simulink library "tenneco_lib"  (R2016b)
settings: Solver=ode45  StartTime=0.0  StopTime=10.0  RelTol=1e-3
undefined symbols (not defined in the file): Com_cntAMBInitTO_c, Com_cntAMBStopTO_c, Com_cntEC1InitTO_c, Com_cntEC1StopTO_c, Com_swAMBRx_c, Com_swEC1Rx_c, Com_swUseSPN108_c, Com_swUseSPN543_c, const, Env_pAmbPDflt_c, Env_pAmbPKOff_c, Env_pAmbPOvrd_c, Env_swAmbPOvrd_c, MSG_INIT_TIMEOUT, MSG_NOT_RECEIVED, MSG_RECEIVED_NOW, MSG_STOP_TIMEOUT
libraries: simulink x19, tenneco_lib x2
(part 4 of 5)

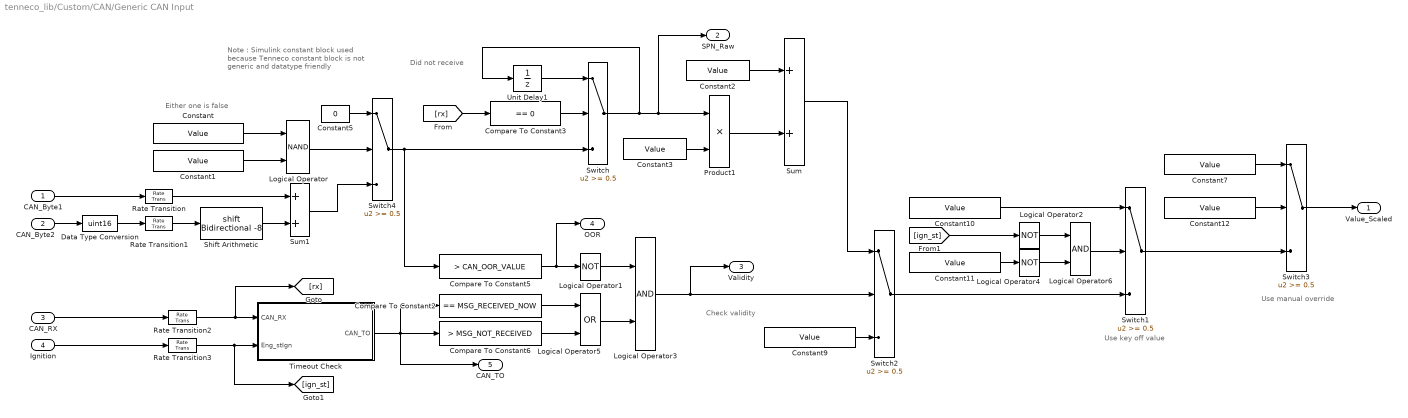
== system tenneco_lib/Custom/CAN/Generic CAN Input ==
  note: Either one is false
  note: Did not receive
  note: Use manual override
  note: Check validity
  note: Use key off value
  note: Note : Simulink constant block used because Tenneco constant block is not generic and datatype friendly
  CAN_Byte1 : Inport  mask(Standard Inport){Port=1}
      mask prompts: Port "Simulink:blkprm_prompts:InOutportPortNum"
      mask help: Provide an input port for subsystems.
      mask TypeOptions Port: Port
  CAN_Byte2 : Inport  Port=2  mask(Standard Inport){Port=2}
      mask prompts: Port "Simulink:blkprm_prompts:InOutportPortNum"
      mask help: Provide an input port for subsystems.
      mask TypeOptions Port: Port
  CAN_RX : Inport  Port=3  mask(Standard Inport){Port=3}
      mask prompts: Port "Simulink:blkprm_prompts:InOutportPortNum"
      mask help: Provide an input port for subsystems.
      mask TypeOptions Port: Port
  Ignition : Inport  Port=4  mask(Standard Inport){Port=4}
      mask prompts: Port "Simulink:blkprm_prompts:InOutportPortNum"
      mask help: Provide an input port for subsystems.
      mask TypeOptions Port: Port
  Compare To Constant2 : simulink/Logic and Bit Operations/Compare To Constant  relop===  const=MSG_RECEIVED_NOW  OutDataTypeStr=boolean
  Compare To Constant3 : simulink/Logic and Bit Operations/Compare To Constant  relop===  const=0  OutDataTypeStr=boolean
  Compare To Constant5 : simulink/Logic and Bit Operations/Compare To Constant  relop=>  const=CAN_OOR_VALUE  OutDataTypeStr=boolean
  Compare To Constant6 : simulink/Logic and Bit Operations/Compare To Constant  relop=>  const=MSG_NOT_RECEIVED  OutDataTypeStr=boolean
  Constant : Constant  Value=Value  mask(Constant){Value=CAN_USE_SW}
      mask prompts: Value "Simulink:blkprm_prompts:ConstConstValue"
      mask help: Output the constant specified by the 'Constant value' parameter. If 'Constant value' is a vector, treat the constant value as a 1-D array.
      mask init: same as tenneco_lib/Sources/Constant
      mask TypeOptions Value: Value
      mask Display: disp(str)
  Constant1 : Constant  Value=Value  mask(Constant){Value=CAN_RECV_SW}
      mask prompts: Value "Simulink:blkprm_prompts:ConstConstValue"
      mask help: Output the constant specified by the 'Constant value' parameter. If 'Constant value' is a vector, treat the constant value as a 1-D array.
      mask init: same as tenneco_lib/Sources/Constant
      mask TypeOptions Value: Value
      mask Display: disp(str)
  Constant10 : Constant  Value=Value  mask(Constant){Value=KEY_OFF_VALUE}
      mask prompts: Value "Simulink:blkprm_prompts:ConstConstValue"
      mask help: Output the constant specified by the 'Constant value' parameter. If 'Constant value' is a vector, treat the constant value as a 1-D array.
      mask init: same as tenneco_lib/Sources/Constant
      mask TypeOptions Value: Value
      mask Display: disp(str)
  Constant11 : Constant  Value=Value  mask(Constant){Value=MAN_OVRD_SW}
      mask prompts: Value "Simulink:blkprm_prompts:ConstConstValue"
      mask help: Output the constant specified by the 'Constant value' parameter. If 'Constant value' is a vector, treat the constant value as a 1-D array.
      mask init: same as tenneco_lib/Sources/Constant
      mask TypeOptions Value: Value
      mask Display: disp(str)
  Constant12 : Constant  Value=Value  mask(Constant){Value=MAN_OVRD_SW}
      mask prompts: Value "Simulink:blkprm_prompts:ConstConstValue"
      mask help: Output the constant specified by the 'Constant value' parameter. If 'Constant value' is a vector, treat the constant value as a 1-D array.
      mask init: same as tenneco_lib/Sources/Constant
      mask TypeOptions Value: Value
      mask Display: disp(str)
  Constant2 : Constant  Value=Value  mask(Constant){Value=OFFSET}
      mask prompts: Value "Simulink:blkprm_prompts:ConstConstValue"
      mask help: Output the constant specified by the 'Constant value' parameter. If 'Constant value' is a vector, treat the constant value as a 1-D array.
      mask init: same as tenneco_lib/Sources/Constant
      mask TypeOptions Value: Value
      mask Display: disp(str)
  Constant3 : Constant  Value=Value  mask(Constant){Value=SLOPE}
      mask prompts: Value "Simulink:blkprm_prompts:ConstConstValue"
      mask help: Output the constant specified by the 'Constant value' parameter. If 'Constant value' is a vector, treat the constant value as a 1-D array.
      mask init: same as tenneco_lib/Sources/Constant
      mask TypeOptions Value: Value
      mask Display: disp(str)
  Constant5 : Constant  Value=0  OutDataTypeStr=Inherit: Inherit via back propagation
  Constant7 : Constant  Value=Value  mask(Constant){Value=MAN_OVRD_VALUE}
      mask prompts: Value "Simulink:blkprm_prompts:ConstConstValue"
      mask help: Output the constant specified by the 'Constant value' parameter. If 'Constant value' is a vector, treat the constant value as a 1-D array.
      mask init: same as tenneco_lib/Sources/Constant
      mask TypeOptions Value: Value
      mask Display: disp(str)
  Constant9 : Constant  Value=Value  mask(Constant){Value=DEFAULT_VALUE}
      mask prompts: Value "Simulink:blkprm_prompts:ConstConstValue"
      mask help: Output the constant specified by the 'Constant value' parameter. If 'Constant value' is a vector, treat the constant value as a 1-D array.
      mask init: same as tenneco_lib/Sources/Constant
      mask TypeOptions Value: Value
      mask Display: disp(str)
  Data Type Conversion : DataTypeConversion  OutDataTypeStr=uint16  mask(Data Type Conversion){OutDataTypeStr=uint16}
      mask prompts: OutDataTypeStr "Simulink:blkprm_prompts:OUTPUT_UNIFIEDDATATYPE"
      mask help: Convert the input to the data type and scaling of the output.
      mask TypeOptions OutDataTypeStr: OutDataTypeStr
  Logical Operator : Logic  Operator=NAND  Inputs=Inputs  AllPortsSameDT=off  OutDataTypeStr=boolean  mask(Logical Operator){Operator=NAND, Inputs=2}
      mask prompts: Operator "Simulink:blkprm_prompts:LogicOperator"; Inputs "Simulink:blkprm_prompts:LogicNumInputPorts"
      mask help: Logical operators. For a single input, operators are applied across the input vector. For multiple inputs, operators are applied across the inputs.
      mask TypeOptions Operator: Operator
      mask TypeOptions Inputs: Inputs
  Logical Operator1 : Logic  Operator=NOT  Inputs=Inputs  AllPortsSameDT=off  OutDataTypeStr=boolean  mask(Logical Operator){Operator=NOT, Inputs=2}
      mask prompts: Operator "Simulink:blkprm_prompts:LogicOperator"; Inputs "Simulink:blkprm_prompts:LogicNumInputPorts"
      mask help: Logical operators. For a single input, operators are applied across the input vector. For multiple inputs, operators are applied across the inputs.
      mask TypeOptions Operator: Operator
      mask TypeOptions Inputs: Inputs
  Logical Operator2 : Logic  Operator=NOT  Inputs=Inputs  AllPortsSameDT=off  OutDataTypeStr=boolean  mask(Logical Operator){Operator=NOT, Inputs=2}
      mask prompts: Operator "Simulink:blkprm_prompts:LogicOperator"; Inputs "Simulink:blkprm_prompts:LogicNumInputPorts"
      mask help: Logical operators. For a single input, operators are applied across the input vector. For multiple inputs, operators are applied across the inputs.
      mask TypeOptions Operator: Operator
      mask TypeOptions Inputs: Inputs
  Logical Operator3 : Logic  Inputs=Inputs  AllPortsSameDT=off  OutDataTypeStr=boolean  mask(Logical Operator){Operator=AND, Inputs=2}
      mask prompts: Operator "Simulink:blkprm_prompts:LogicOperator"; Inputs "Simulink:blkprm_prompts:LogicNumInputPorts"
      mask help: Logical operators. For a single input, operators are applied across the input vector. For multiple inputs, operators are applied across the inputs.
      mask TypeOptions Operator: Operator
      mask TypeOptions Inputs: Inputs
  Logical Operator4 : Logic  Operator=NOT  Inputs=Inputs  AllPortsSameDT=off  OutDataTypeStr=boolean  mask(Logical Operator){Operator=NOT, Inputs=2}
      mask prompts: Operator "Simulink:blkprm_prompts:LogicOperator"; Inputs "Simulink:blkprm_prompts:LogicNumInputPorts"
      mask help: Logical operators. For a single input, operators are applied across the input vector. For multiple inputs, operators are applied across the inputs.
      mask TypeOptions Operator: Operator
      mask TypeOptions Inputs: Inputs
  Logical Operator5 : Logic  Operator=OR  Inputs=Inputs  AllPortsSameDT=off  OutDataTypeStr=boolean  mask(Logical Operator){Operator=OR, Inputs=2}
      mask prompts: Operator "Simulink:blkprm_prompts:LogicOperator"; Inputs "Simulink:blkprm_prompts:LogicNumInputPorts"
      mask help: Logical operators. For a single input, operators are applied across the input vector. For multiple inputs, operators are applied across the inputs.
      mask TypeOptions Operator: Operator
      mask TypeOptions Inputs: Inputs
  Logical Operator6 : Logic  Inputs=Inputs  AllPortsSameDT=off  OutDataTypeStr=boolean  mask(Logical Operator){Operator=AND, Inputs=2}
      mask prompts: Operator "Simulink:blkprm_prompts:LogicOperator"; Inputs "Simulink:blkprm_prompts:LogicNumInputPorts"
      mask help: Logical operators. For a single input, operators are applied across the input vector. For multiple inputs, operators are applied across the inputs.
      mask TypeOptions Operator: Operator
      mask TypeOptions Inputs: Inputs
  Product1 : Product  Inputs=**  InputSameDT=on  mask(Product){Inputs=**}
      mask prompts: Inputs "List of signs:"
      mask help:
      | Multiply or divide inputs.  Specify one of the following:
      |  a) * or / for each input port. For example, **/* performs the operation 'u1*u2/u3*u4'.
      |  b) scalar specifies the number of input ports to be multiplied.
      mask TypeOptions Inputs: Inputs
  Rate Transition{,1..3} (4 alike) : RateTransition  OutPortSampleTime=RATE
  Shift Arithmetic : ArithShift  BitShiftNumber=-8
  Sum : Sum  InputSameDT=on  mask(Sum){Inputs=++}
      mask prompts: Inputs "Simulink:blkprm_prompts:SumListofSigns"
      mask help:
      | Add or subtract inputs.  Specify one of the following:
      | a) character vector containing + or - for each input port, | for spacer between ports (e.g. ++|-|++)
      | b) scalar, >= 1, specifies the number of input ports to be summed.
      | When there is only one input port, add or subtract elements over all dimensions or one specified dimension
      mask TypeOptions Inputs: Inputs
  Sum1 : Sum  InputSameDT=on  mask(Sum){Inputs=++}
      mask prompts: Inputs "Simulink:blkprm_prompts:SumListofSigns"
      mask help:
      | Add or subtract inputs.  Specify one of the following:
      | a) character vector containing + or - for each input port, | for spacer between ports (e.g. ++|-|++)
      | b) scalar, >= 1, specifies the number of input ports to be summed.
      | When there is only one input port, add or subtract elements over all dimensions or one specified dimension
      mask TypeOptions Inputs: Inputs
  Switch : Switch  Threshold=0.5  mask(Switch){}
      mask help: Pass through input 1 when input 2 satisfies the selected criterion; otherwise, pass through input 3. The inputs are numbered top to bottom (or left to right). The first and third input ports are data ports, and the second input port is the control port. The criteria for control port 2 are u2 >= Threshold (0.5).
  Switch1 : Switch  Threshold=0.5  mask(Switch){}
      mask help: Pass through input 1 when input 2 satisfies the selected criterion; otherwise, pass through input 3. The inputs are numbered top to bottom (or left to right). The first and third input ports are data ports, and the second input port is the control port. The criteria for control port 2 are u2 >= Threshold (0.5).
  Switch2 : Switch  Threshold=0.5  mask(Switch){}
      mask help: Pass through input 1 when input 2 satisfies the selected criterion; otherwise, pass through input 3. The inputs are numbered top to bottom (or left to right). The first and third input ports are data ports, and the second input port is the control port. The criteria for control port 2 are u2 >= Threshold (0.5).
  Switch3 : Switch  Threshold=0.5  mask(Switch){}
      mask help: Pass through input 1 when input 2 satisfies the selected criterion; otherwise, pass through input 3. The inputs are numbered top to bottom (or left to right). The first and third input ports are data ports, and the second input port is the control port. The criteria for control port 2 are u2 >= Threshold (0.5).
  Switch4 : Switch  Threshold=0.5  mask(Switch){}
      mask help: Pass through input 1 when input 2 satisfies the selected criterion; otherwise, pass through input 3. The inputs are numbered top to bottom (or left to right). The first and third input ports are data ports, and the second input port is the control port. The criteria for control port 2 are u2 >= Threshold (0.5).
  Timeout Check : Subsystem
  Unit Delay1 : UnitDelay  InitialCondition=InitialCondition  SampleTime=-1  mask(Unit Delay){InitialCondition=0}
      mask prompts: InitialCondition "Simulink:blkprm_prompts:DelayBlkInitCond"
      mask help: Sample and hold with one sample period delay.
      mask TypeOptions InitialCondition: InitialCondition
  Value_Scaled : Outport  mask(Standard Outport){Port=1}
      mask prompts: Port "Simulink:blkprm_prompts:InOutportPortNum"
      mask help: Provide an output port for subsystems.
      mask TypeOptions Port: Port
  SPN_Raw : Outport  Port=2  mask(Standard Outport){Port=2}
      mask prompts: Port "Simulink:blkprm_prompts:InOutportPortNum"
      mask help: Provide an output port for subsystems.
      mask TypeOptions Port: Port
  Validity : Outport  Port=3  mask(Standard Outport){Port=3}
      mask prompts: Port "Simulink:blkprm_prompts:InOutportPortNum"
      mask help: Provide an output port for subsystems.
      mask TypeOptions Port: Port
  OOR : Outport  Port=4  mask(Standard Outport){Port=4}
      mask prompts: Port "Simulink:blkprm_prompts:InOutportPortNum"
      mask help: Provide an output port for subsystems.
      mask TypeOptions Port: Port
  CAN_TO : Outport  Port=5  mask(Standard Outport){Port=5}
      mask prompts: Port "Simulink:blkprm_prompts:InOutportPortNum"
      mask help: Provide an output port for subsystems.
      mask TypeOptions Port: Port
  wires:
  Constant1/1 -> Logical Operator/2
  Data Type Conversion/1 -> Rate Transition1/1
  CAN_Byte1/1 -> Rate Transition/1
  CAN_Byte2/1 -> Data Type Conversion/1
  Rate Transition/1 -> Sum1/1
  Rate Transition1/1 -> Shift Arithmetic/1
  Shift Arithmetic/1 -> Sum1/2
  Sum1/1 -> Switch4/3
  Constant5/1 -> Switch4/1
  Logical Operator/1 -> Switch4/2
  Constant/1 -> Logical Operator/1
  [rx] -> Compare To Constant3/1
  Switch4/1 -> Switch/3, Compare To Constant5/1
  Unit Delay1/1 -> Switch/1
  Compare To Constant3/1 -> Switch/2
  Switch/1 -> SPN_Raw/1, Product1/1, Unit Delay1/1
  Rate Transition3/1 -> Timeout Check/2(Eng_stIgn), [ign_st]
  Rate Transition2/1 -> [rx], Timeout Check/1(CAN_RX)
  Constant3/1 -> Product1/2
  Ignition/1 -> Rate Transition3/1
  CAN_RX/1 -> Rate Transition2/1
  Constant7/1 -> Switch3/1
  Constant12/1 -> Switch3/2
  Compare To Constant6/1 -> Logical Operator5/2
  Compare To Constant2/1 -> Logical Operator5/1
  Compare To Constant5/1 -> OOR/1, Logical Operator1/1
  Logical Operator3/1 -> Switch2/2, Validity/1
  Switch3/1 -> Value_Scaled/1
  [ign_st] -> Logical Operator2/1
  Logical Operator2/1 -> Logical Operator6/1
  Constant11/1 -> Logical Operator4/1
  Constant10/1 -> Switch1/1
  Logical Operator6/1 -> Switch1/2
  Switch1/1 -> Switch3/3
  Constant9/1 -> Switch2/3
  Sum/1 -> Switch2/1
  Logical Operator1/1 -> Logical Operator3/1
  Logical Operator5/1 -> Logical Operator3/2
  Timeout Check/1(CAN_TO) -> Compare To Constant6/1, Compare To Constant2/1, CAN_TO/1
  Switch2/1 -> Switch1/3
  Logical Operator4/1 -> Logical Operator6/2
  Constant2/1 -> Sum/1
  Product1/1 -> Sum/2

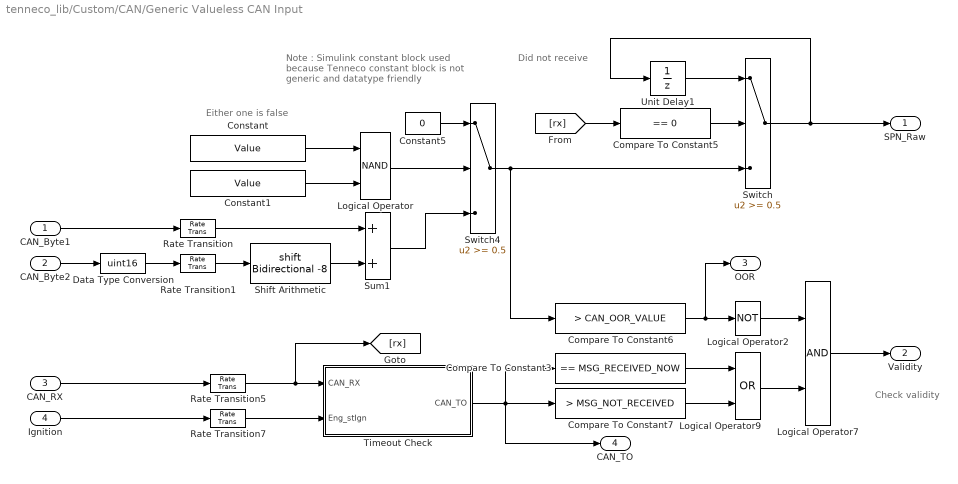
== system tenneco_lib/Custom/CAN/Generic Valueless CAN Input ==
  note: Either one is false
  note: Did not receive
  note: Check validity
  note: Note : Simulink constant block used because Tenneco constant block is not generic and datatype friendly
  CAN_Byte1 : Inport  mask(Standard Inport){Port=1}
      mask prompts: Port "Simulink:blkprm_prompts:InOutportPortNum"
      mask help: Provide an input port for subsystems.
      mask TypeOptions Port: Port
  CAN_Byte2 : Inport  Port=2  mask(Standard Inport){Port=2}
      mask prompts: Port "Simulink:blkprm_prompts:InOutportPortNum"
      mask help: Provide an input port for subsystems.
      mask TypeOptions Port: Port
  CAN_RX : Inport  Port=3  mask(Standard Inport){Port=3}
      mask prompts: Port "Simulink:blkprm_prompts:InOutportPortNum"
      mask help: Provide an input port for subsystems.
      mask TypeOptions Port: Port
  Ignition : Inport  Port=4  mask(Standard Inport){Port=4}
      mask prompts: Port "Simulink:blkprm_prompts:InOutportPortNum"
      mask help: Provide an input port for subsystems.
      mask TypeOptions Port: Port
  Compare To Constant3 : simulink/Logic and Bit Operations/Compare To Constant  relop===  const=MSG_RECEIVED_NOW  OutDataTypeStr=boolean
  Compare To Constant5 : simulink/Logic and Bit Operations/Compare To Constant  relop===  const=0  OutDataTypeStr=boolean
  Compare To Constant6 : simulink/Logic and Bit Operations/Compare To Constant  relop=>  const=CAN_OOR_VALUE  OutDataTypeStr=boolean
  Compare To Constant7 : simulink/Logic and Bit Operations/Compare To Constant  relop=>  const=MSG_NOT_RECEIVED  OutDataTypeStr=boolean
  Constant : Constant  Value=Value  mask(Constant){Value=CAN_USE_SW}
      mask prompts: Value "Simulink:blkprm_prompts:ConstConstValue"
      mask help: Output the constant specified by the 'Constant value' parameter. If 'Constant value' is a vector, treat the constant value as a 1-D array.
      mask init: same as tenneco_lib/Sources/Constant
      mask TypeOptions Value: Value
      mask Display: disp(str)
  Constant1 : Constant  Value=Value  mask(Constant){Value=CAN_RECV_SW}
      mask prompts: Value "Simulink:blkprm_prompts:ConstConstValue"
      mask help: Output the constant specified by the 'Constant value' parameter. If 'Constant value' is a vector, treat the constant value as a 1-D array.
      mask init: same as tenneco_lib/Sources/Constant
      mask TypeOptions Value: Value
      mask Display: disp(str)
  Constant5 : Constant  Value=0  OutDataTypeStr=Inherit: Inherit via back propagation
  Data Type Conversion : DataTypeConversion  OutDataTypeStr=uint16  mask(Data Type Conversion){OutDataTypeStr=uint16}
      mask prompts: OutDataTypeStr "Simulink:blkprm_prompts:OUTPUT_UNIFIEDDATATYPE"
      mask help: Convert the input to the data type and scaling of the output.
      mask TypeOptions OutDataTypeStr: OutDataTypeStr
  Logical Operator : Logic  Operator=NAND  Inputs=Inputs  AllPortsSameDT=off  OutDataTypeStr=boolean  mask(Logical Operator){Operator=NAND, Inputs=2}
      mask prompts: Operator "Simulink:blkprm_prompts:LogicOperator"; Inputs "Simulink:blkprm_prompts:LogicNumInputPorts"
      mask help: Logical operators. For a single input, operators are applied across the input vector. For multiple inputs, operators are applied across the inputs.
      mask TypeOptions Operator: Operator
      mask TypeOptions Inputs: Inputs
  Logical Operator2 : Logic  Operator=NOT  Inputs=Inputs  AllPortsSameDT=off  OutDataTypeStr=boolean  mask(Logical Operator){Operator=NOT, Inputs=2}
      mask prompts: Operator "Simulink:blkprm_prompts:LogicOperator"; Inputs "Simulink:blkprm_prompts:LogicNumInputPorts"
      mask help: Logical operators. For a single input, operators are applied across the input vector. For multiple inputs, operators are applied across the inputs.
      mask TypeOptions Operator: Operator
      mask TypeOptions Inputs: Inputs
  Logical Operator7 : Logic  Inputs=Inputs  AllPortsSameDT=off  OutDataTypeStr=boolean  mask(Logical Operator){Operator=AND, Inputs=2}
      mask prompts: Operator "Simulink:blkprm_prompts:LogicOperator"; Inputs "Simulink:blkprm_prompts:LogicNumInputPorts"
      mask help: Logical operators. For a single input, operators are applied across the input vector. For multiple inputs, operators are applied across the inputs.
      mask TypeOptions Operator: Operator
      mask TypeOptions Inputs: Inputs
  Logical Operator9 : Logic  Operator=OR  Inputs=Inputs  AllPortsSameDT=off  OutDataTypeStr=boolean  mask(Logical Operator){Operator=OR, Inputs=2}
      mask prompts: Operator "Simulink:blkprm_prompts:LogicOperator"; Inputs "Simulink:blkprm_prompts:LogicNumInputPorts"
      mask help: Logical operators. For a single input, operators are applied across the input vector. For multiple inputs, operators are applied across the inputs.
      mask TypeOptions Operator: Operator
      mask TypeOptions Inputs: Inputs
  Rate Transition{,1,5,7} (4 alike) : RateTransition  OutPortSampleTime=RATE
  Shift Arithmetic : ArithShift  BitShiftNumber=-8
  Sum1 : Sum  InputSameDT=on  mask(Sum){Inputs=++}
      mask prompts: Inputs "Simulink:blkprm_prompts:SumListofSigns"
      mask help:
      | Add or subtract inputs.  Specify one of the following:
      | a) character vector containing + or - for each input port, | for spacer between ports (e.g. ++|-|++)
      | b) scalar, >= 1, specifies the number of input ports to be summed.
      | When there is only one input port, add or subtract elements over all dimensions or one specified dimension
      mask TypeOptions Inputs: Inputs
  Switch : Switch  Threshold=0.5  mask(Switch){}
      mask help: Pass through input 1 when input 2 satisfies the selected criterion; otherwise, pass through input 3. The inputs are numbered top to bottom (or left to right). The first and third input ports are data ports, and the second input port is the control port. The criteria for control port 2 are u2 >= Threshold (0.5).
  Switch4 : Switch  Threshold=0.5  mask(Switch){}
      mask help: Pass through input 1 when input 2 satisfies the selected criterion; otherwise, pass through input 3. The inputs are numbered top to bottom (or left to right). The first and third input ports are data ports, and the second input port is the control port. The criteria for control port 2 are u2 >= Threshold (0.5).
  Timeout Check : Subsystem
  Unit Delay1 : UnitDelay  InitialCondition=InitialCondition  SampleTime=-1  mask(Unit Delay){InitialCondition=0}
      mask prompts: InitialCondition "Simulink:blkprm_prompts:DelayBlkInitCond"
      mask help: Sample and hold with one sample period delay.
      mask TypeOptions InitialCondition: InitialCondition
  SPN_Raw : Outport  mask(Standard Outport){Port=1}
      mask prompts: Port "Simulink:blkprm_prompts:InOutportPortNum"
      mask help: Provide an output port for subsystems.
      mask TypeOptions Port: Port
  Validity : Outport  Port=2  mask(Standard Outport){Port=2}
      mask prompts: Port "Simulink:blkprm_prompts:InOutportPortNum"
      mask help: Provide an output port for subsystems.
      mask TypeOptions Port: Port
  OOR : Outport  Port=3  mask(Standard Outport){Port=3}
      mask prompts: Port "Simulink:blkprm_prompts:InOutportPortNum"
      mask help: Provide an output port for subsystems.
      mask TypeOptions Port: Port
  CAN_TO : Outport  Port=4  mask(Standard Outport){Port=4}
      mask prompts: Port "Simulink:blkprm_prompts:InOutportPortNum"
      mask help: Provide an output port for subsystems.
      mask TypeOptions Port: Port
  wires:
  CAN_Byte2/1 -> Data Type Conversion/1
  Constant1/1 -> Logical Operator/2
  Data Type Conversion/1 -> Rate Transition1/1
  CAN_Byte1/1 -> Rate Transition/1
  Rate Transition/1 -> Sum1/1
  Rate Transition1/1 -> Shift Arithmetic/1
  Shift Arithmetic/1 -> Sum1/2
  Sum1/1 -> Switch4/3
  Constant5/1 -> Switch4/1
  Logical Operator/1 -> Switch4/2
  Constant/1 -> Logical Operator/1
  [rx] -> Compare To Constant5/1
  Switch4/1 -> Switch/3, Compare To Constant6/1
  Unit Delay1/1 -> Switch/1
  Compare To Constant5/1 -> Switch/2
  Switch/1 -> SPN_Raw/1, Unit Delay1/1
  Rate Transition7/1 -> Timeout Check/2(Eng_stIgn)
  Rate Transition5/1 -> [rx], Timeout Check/1(CAN_RX)
  Ignition/1 -> Rate Transition7/1
  CAN_RX/1 -> Rate Transition5/1
  Compare To Constant7/1 -> Logical Operator9/2
  Compare To Constant3/1 -> Logical Operator9/1
  Compare To Constant6/1 -> Logical Operator2/1, OOR/1
  Logical Operator7/1 -> Validity/1
  Logical Operator2/1 -> Logical Operator7/1
  Logical Operator9/1 -> Logical Operator7/2
  Timeout Check/1(CAN_TO) -> Compare To Constant7/1, Compare To Constant3/1, CAN_TO/1

== system tenneco_lib/Custom/CAN/Timeout Check ==
  Input Signal : Inport  mask(Standard Inport){Port=1}
      mask prompts: Port "Simulink:blkprm_prompts:InOutportPortNum"
      mask help: Provide an input port for subsystems.
      mask TypeOptions Port: Port
  Enable : Inport  Port=2  mask(Standard Inport){Port=2}
      mask prompts: Port "Simulink:blkprm_prompts:InOutportPortNum"
      mask help: Provide an input port for subsystems.
      mask TypeOptions Port: Port
  Init Timeout Limit : Inport  Port=3  mask(Standard Inport){Port=3}
      mask prompts: Port "Simulink:blkprm_prompts:InOutportPortNum"
      mask help: Provide an input port for subsystems.
      mask TypeOptions Port: Port
  Stop Timeout Limit : Inport  Port=4  mask(Standard Inport){Port=4}
      mask prompts: Port "Simulink:blkprm_prompts:InOutportPortNum"
      mask help: Provide an input port for subsystems.
      mask TypeOptions Port: Port
  Constant : Constant  Value=Value  mask(Constant){Value=MSG_NOT_RECEIVED}
      mask prompts: Value "Simulink:blkprm_prompts:ConstConstValue"
      mask help: Output the constant specified by the 'Constant value' parameter. If 'Constant value' is a vector, treat the constant value as a 1-D array.
      mask init: same as tenneco_lib/Sources/Constant
      mask TypeOptions Value: Value
      mask Display: disp(str)
  Data Type Conversion1 : DataTypeConversion  OutDataTypeStr=boolean  mask(Data Type Conversion){OutDataTypeStr=boolean}
      mask prompts: OutDataTypeStr "Simulink:blkprm_prompts:OUTPUT_UNIFIEDDATATYPE"
      mask help: Convert the input to the data type and scaling of the output.
      mask TypeOptions OutDataTypeStr: OutDataTypeStr
  Data Type Conversion2 : DataTypeConversion  OutDataTypeStr=uint8  mask(Data Type Conversion){OutDataTypeStr=uint8}
      mask prompts: OutDataTypeStr "Simulink:blkprm_prompts:OUTPUT_UNIFIEDDATATYPE"
      mask help: Convert the input to the data type and scaling of the output.
      mask TypeOptions OutDataTypeStr: OutDataTypeStr
  Data Type Conversion3 : DataTypeConversion  OutDataTypeStr=uint8  mask(Data Type Conversion){OutDataTypeStr=uint8}
      mask prompts: OutDataTypeStr "Simulink:blkprm_prompts:OUTPUT_UNIFIEDDATATYPE"
      mask help: Convert the input to the data type and scaling of the output.
      mask TypeOptions OutDataTypeStr: OutDataTypeStr
  Data Type Conversion4 : DataTypeConversion  OutDataTypeStr=boolean  mask(Data Type Conversion){OutDataTypeStr=boolean}
      mask prompts: OutDataTypeStr "Simulink:blkprm_prompts:OUTPUT_UNIFIEDDATATYPE"
      mask help: Convert the input to the data type and scaling of the output.
      mask TypeOptions OutDataTypeStr: OutDataTypeStr
  Switch : Switch  Threshold=0.5  mask(Switch){}
      mask help: Pass through input 1 when input 2 satisfies the selected criterion; otherwise, pass through input 3. The inputs are numbered top to bottom (or left to right). The first and third input ports are data ports, and the second input port is the control port. The criteria for control port 2 are u2 >= Threshold (0.5).
  Timeout Check : Subsystem  TreatAsAtomicUnit=on
  Timeout Code : Outport  mask(Standard Outport){Port=1}
      mask prompts: Port "Simulink:blkprm_prompts:InOutportPortNum"
      mask help: Provide an output port for subsystems.
      mask TypeOptions Port: Port
  wires:
  Constant/1 -> Switch/3
  Timeout Check/1(Timeout Code) -> Switch/1
  Switch/1 -> Timeout Code/1
  Input Signal/1 -> Data Type Conversion1/1
  Enable/1 -> Data Type Conversion4/1
  Data Type Conversion1/1 -> Timeout Check/1(Input Signal)
  Data Type Conversion4/1 -> [fxn_enable], Timeout Check/Enable
  [fxn_enable] -> Switch/2
  Data Type Conversion2/1 -> Timeout Check/2(Init Timeout Limit)
  Data Type Conversion3/1 -> Timeout Check/3(Stop Timeout Limit)
  Init Timeout Limit/1 -> Data Type Conversion2/1
  Stop Timeout Limit/1 -> Data Type Conversion3/1

== system tenneco_lib/Custom/Logical/Latch ==
  Set : Inport  mask(Standard Inport){Port=1}
      mask prompts: Port "Simulink:blkprm_prompts:InOutportPortNum"
      mask help: Provide an input port for subsystems.
      mask TypeOptions Port: Port
  Reset : Inport  Port=2  mask(Standard Inport){Port=2}
      mask prompts: Port "Simulink:blkprm_prompts:InOutportPortNum"
      mask help: Provide an input port for subsystems.
      mask TypeOptions Port: Port
  Constant : Constant  Value=Value  mask(Constant){Value=INIT}
      mask prompts: Value "Simulink:blkprm_prompts:ConstConstValue"
      mask help: Output the constant specified by the 'Constant value' parameter. If 'Constant value' is a vector, treat the constant value as a 1-D array.
      mask init:
      | blkName = gcb;
      | 
      | str = ['C']; %default
      | 
      | const_str = get_param(blkName, 'Value');
      | const_val = str2num(const_str);
      | 
      | if isempty(const_val) %#ok<ST2NM>
      |     %Expression/Variable
      |     str = [strtrim(const_str)];
      | else
      |     if length(const_val) == 1 
      |         if Simulink.data.isSupportedEnumClass(class(const_val))
      |             % Special Handling for Enumerations
      |             if Simulink.data.getEnumTypeInfo(class(const_val), 'AddClassNameToEnumNames')
      |                 str = [strtrim(const_str)];
      |             else
      |                 str = [char(const_val)];
      |             end
      |         elseif(isfloat(const_val) || isinteger(const_val)) 
      |                 str = [num2str(const_val)];
      |         end
      |     end
      | end
      mask TypeOptions Value: Value
      mask Display: disp(str)
  Constant5 : Constant  Value=0  OutDataTypeStr=Inherit: Inherit via back propagation
  Data Type Conversion1 : DataTypeConversion  OutDataTypeStr=boolean  mask(Data Type Conversion){OutDataTypeStr=boolean}
      mask prompts: OutDataTypeStr "Simulink:blkprm_prompts:OUTPUT_UNIFIEDDATATYPE"
      mask help: Convert the input to the data type and scaling of the output.
      mask TypeOptions OutDataTypeStr: OutDataTypeStr
  Logical Operator1 : Logic  Operator=OR  Inputs=Inputs  AllPortsSameDT=off  OutDataTypeStr=boolean  mask(Logical Operator){Operator=OR, Inputs=2}
      mask prompts: Operator "Simulink:blkprm_prompts:LogicOperator"; Inputs "Simulink:blkprm_prompts:LogicNumInputPorts"
      mask help: Logical operators. For a single input, operators are applied across the input vector. For multiple inputs, operators are applied across the inputs.
      mask TypeOptions Operator: Operator
      mask TypeOptions Inputs: Inputs
  Logical Operator2 : Logic  Operator=OR  Inputs=Inputs  AllPortsSameDT=off  OutDataTypeStr=boolean  mask(Logical Operator){Operator=OR, Inputs=2}
      mask prompts: Operator "Simulink:blkprm_prompts:LogicOperator"; Inputs "Simulink:blkprm_prompts:LogicNumInputPorts"
      mask help: Logical operators. For a single input, operators are applied across the input vector. For multiple inputs, operators are applied across the inputs.
      mask TypeOptions Operator: Operator
      mask TypeOptions Inputs: Inputs
  Switch1 : Switch  Threshold=0.5  mask(Switch){}
      mask help: Pass through input 1 when input 2 satisfies the selected criterion; otherwise, pass through input 3. The inputs are numbered top to bottom (or left to right). The first and third input ports are data ports, and the second input port is the control port. The criteria for control port 2 are u2 >= Threshold (0.5).
  Unit Delay : UnitDelay  InitialCondition=InitialCondition  SampleTime=-1  mask(Unit Delay){InitialCondition=1}
      mask prompts: InitialCondition "Simulink:blkprm_prompts:DelayBlkInitCond"
      mask help: Sample and hold with one sample period delay.
      mask TypeOptions InitialCondition: InitialCondition
  Unit Delay1 : UnitDelay  InitialCondition=InitialCondition  SampleTime=-1  mask(Unit Delay){InitialCondition=0}
      mask prompts: InitialCondition "Simulink:blkprm_prompts:DelayBlkInitCond"
      mask help: Sample and hold with one sample period delay.
      mask TypeOptions InitialCondition: InitialCondition
  Out : Outport  mask(Standard Outport){Port=1}
      mask prompts: Port "Simulink:blkprm_prompts:InOutportPortNum"
      mask help: Provide an output port for subsystems.
      mask TypeOptions Port: Port
  wires:
  Constant/1 -> Switch1/1
  Logical Operator2/1 -> Switch1/2
  Unit Delay/1 -> Logical Operator2/1
  Constant5/1 -> Unit Delay/1
  Reset/1 -> Logical Operator2/2
  Logical Operator1/1 -> Switch1/3
  Set/1 -> Logical Operator1/1
  Switch1/1 -> Unit Delay1/1, Data Type Conversion1/1
  Data Type Conversion1/1 -> Out/1
  Unit Delay1/1 -> Logical Operator1/2

== system tenneco_lib/Custom/Math/Divide by zero protection ==
  U1 : Inport
  U2 : Inport  Port=2
  If Action Subsystem1 : Subsystem  TreatAsAtomicUnit=on
  If Action Subsystem2 : Subsystem  TreatAsAtomicUnit=on
  If1 : If  NumInputs=2  IfExpression=u2 ~= 0  mask(If Block){NumInputs=2, IfExpression=u2 ~= 0, ElseIfExpressions=, ShowElse=on}
      mask prompts: NumInputs "Simulink:blkprm_prompts:IfNumInputs"; IfExpression "Simulink:blkprm_prompts:IfCondition"; ElseIfExpressions "Simulink:blkprm_prompts:ElseIfConds"; ShowElse "Simulink:blkprm_prompts:IfShowElse"
      mask help:
      | IF expression
      |     Run the Action Subsystem connected to 1st output port
      | ELSEIF expression
      |     Run the Action Subsystem connected to 2nd output port
      | ELSE
      |     Run the Action Subsystem connected to last output port
      | END
      | The number of Elseif output ports in the block is equal to the
      | number of comma-separated Elseif expressions entered in the dialog.
      | The If and Elseif expressions can use these MATLAB operators:
      |     <, <=, ==, ~=, >, >=, &, |, ~, (  ), unary-minus
      | on the input port signals named u1, u2, u3, etc.
      mask TypeOptions NumInputs: NumInputs
      mask TypeOptions IfExpression: IfExpression
      mask TypeOptions ElseIfExpressions: ElseIfExpressions
      mask TypeOptions ShowElse: ShowElse
  Merge1 : Merge  Inputs=Inputs  InitialOutput=InitialOutput  mask(Merge){Inputs=2, InitialOutput=[]}
      mask prompts: Inputs "Simulink:blkprm_prompts:MergeNumInputs"; InitialOutput "Simulink:blkprm_prompts:MergeInitOutput"
      mask help: Merge the input signals into a single output signal whose initial value is specified by the 'Initial output' parameter. If 'Initial output' is empty, the Merge block outputs the initial output of one of its driving blocks.
      mask TypeOptions Inputs: Inputs
      mask TypeOptions InitialOutput: InitialOutput
  Y : Outport
  wires:
  Merge1/1 -> Y/1
  If Action Subsystem2/1(Out1) -> Merge1/2
  If Action Subsystem1/1(Out1) -> Merge1/1
  If1/2 -> If Action Subsystem2/Action
  If1/1 -> If Action Subsystem1/Action
  U2/1 -> If Action Subsystem1/2(In2), If1/2
  U1/1 -> If Action Subsystem1/1(In1), If1/1

== system tenneco_lib/Custom/Math/Time_Based_Rate_Limiter ==
  Input : Inport  mask(Standard Inport){Port=1}
      mask prompts: Port "Simulink:blkprm_prompts:InOutportPortNum"
      mask help: Provide an input port for subsystems.
      mask TypeOptions Port: Port
  Rise_Time : Inport  Port=2  mask(Standard Inport){Port=2}
      mask prompts: Port "Simulink:blkprm_prompts:InOutportPortNum"
      mask help: Provide an input port for subsystems.
      mask TypeOptions Port: Port
  Fall_Time : Inport  Port=3  mask(Standard Inport){Port=3}
      mask prompts: Port "Simulink:blkprm_prompts:InOutportPortNum"
      mask help: Provide an input port for subsystems.
      mask TypeOptions Port: Port
  Compare To Constant : simulink/Logic and Bit Operations/Compare To Constant  relop=>=  const=0  OutDataTypeStr=boolean
  First_Order_System : Subsystem
  Sum : Sum  Inputs=+-  InputSameDT=on  mask(Sum){Inputs=+-}
      mask prompts: Inputs "Simulink:blkprm_prompts:SumListofSigns"
      mask help:
      | Add or subtract inputs.  Specify one of the following:
      | a) character vector containing + or - for each input port, | for spacer between ports (e.g. ++|-|++)
      | b) scalar, >= 1, specifies the number of input ports to be summed.
      | When there is only one input port, add or subtract elements over all dimensions or one specified dimension
      mask TypeOptions Inputs: Inputs
  Switch : Switch  Threshold=0.5  mask(Switch){}
      mask help: Pass through input 1 when input 2 satisfies the selected criterion; otherwise, pass through input 3. The inputs are numbered top to bottom (or left to right). The first and third input ports are data ports, and the second input port is the control port. The criteria for control port 2 are u2 >= Threshold (0.5).
  Unit Delay : UnitDelay  InitialCondition=InitialCondition  SampleTime=-1  mask(Unit Delay){InitialCondition=0}
      mask prompts: InitialCondition "Simulink:blkprm_prompts:DelayBlkInitCond"
      mask help: Sample and hold with one sample period delay.
      mask TypeOptions InitialCondition: InitialCondition
  Output : Outport  mask(Standard Outport){Port=1}
      mask prompts: Port "Simulink:blkprm_prompts:InOutportPortNum"
      mask help: Provide an output port for subsystems.
      mask TypeOptions Port: Port
  wires:
  Compare To Constant/1 -> Switch/2
  Switch/1 -> First_Order_System/2(Tau)
  Rise_Time/1 -> Switch/1
  Fall_Time/1 -> Switch/3
  Sum/1 -> Compare To Constant/1
  Unit Delay/1 -> Sum/2
  First_Order_System/1(Output) -> Output/1, Unit Delay/1
  Input/1 -> First_Order_System/1(Input), Sum/1

== system tenneco_lib/Custom/Timers/Delay_Time ==
  condition : Inport  mask(Standard Inport){Port=1}
      mask prompts: Port "Simulink:blkprm_prompts:InOutportPortNum"
      mask help: Provide an input port for subsystems.
      mask TypeOptions Port: Port
  delay_t : Inport  Port=2  mask(Standard Inport){Port=2}
      mask prompts: Port "Simulink:blkprm_prompts:InOutportPortNum"
      mask help: Provide an input port for subsystems.
      mask TypeOptions Port: Port
  step_time : Inport  Port=3  mask(Standard Inport){Port=3}
      mask prompts: Port "Simulink:blkprm_prompts:InOutportPortNum"
      mask help: Provide an input port for subsystems.
      mask TypeOptions Port: Port
  Constant5 : Constant  Value=0  OutDataTypeStr=Inherit: Inherit via back propagation
  Relational Operator : RelationalOperator  Operator=>  OutDataTypeStr=boolean  RndMeth=Nearest  mask(Relational Operator){Operator=>}
      mask prompts: Operator "Simulink:blkprm_prompts:RelopOperator"
      mask help: Applies the selected relational operator to the inputs and outputs the result. The top (or left) input corresponds to the first operand.
      mask TypeOptions Operator: Operator
  Sum : Sum  InputSameDT=on  mask(Sum){Inputs=++}
      mask prompts: Inputs "Simulink:blkprm_prompts:SumListofSigns"
      mask help:
      | Add or subtract inputs.  Specify one of the following:
      | a) character vector containing + or - for each input port, | for spacer between ports (e.g. ++|-|++)
      | b) scalar, >= 1, specifies the number of input ports to be summed.
      | When there is only one input port, add or subtract elements over all dimensions or one specified dimension
      mask TypeOptions Inputs: Inputs
  Switch1 : Switch  Threshold=0.5  mask(Switch){}
      mask help: Pass through input 1 when input 2 satisfies the selected criterion; otherwise, pass through input 3. The inputs are numbered top to bottom (or left to right). The first and third input ports are data ports, and the second input port is the control port. The criteria for control port 2 are u2 >= Threshold (0.5).
  Unit Delay : UnitDelay  InitialCondition=InitialCondition  SampleTime=-1  mask(Unit Delay){InitialCondition=0}
      mask prompts: InitialCondition "Simulink:blkprm_prompts:DelayBlkInitCond"
      mask help: Sample and hold with one sample period delay.
      mask TypeOptions InitialCondition: InitialCondition
  delay_act : Outport  mask(Standard Outport){Port=1}
      mask prompts: Port "Simulink:blkprm_prompts:InOutportPortNum"
      mask help: Provide an output port for subsystems.
      mask TypeOptions Port: Port
  wires:
  Unit Delay/1 -> Sum/1
  step_time/1 -> Sum/2
  Constant5/1 -> Switch1/3
  delay_t/1 -> Relational Operator/2
  Relational Operator/1 -> delay_act/1
  condition/1 -> Switch1/2
  Switch1/1 -> Unit Delay/1, Relational Operator/1
  Sum/1 -> Switch1/1

== system tenneco_lib/Custom/Timers/Hold_Time ==
  condition : Inport  mask(Standard Inport){Port=1}
      mask prompts: Port "Simulink:blkprm_prompts:InOutportPortNum"
      mask help: Provide an input port for subsystems.
      mask TypeOptions Port: Port
  hold_t : Inport  Port=2  mask(Standard Inport){Port=2}
      mask prompts: Port "Simulink:blkprm_prompts:InOutportPortNum"
      mask help: Provide an input port for subsystems.
      mask TypeOptions Port: Port
  step_time : Inport  Port=3  mask(Standard Inport){Port=3}
      mask prompts: Port "Simulink:blkprm_prompts:InOutportPortNum"
      mask help: Provide an input port for subsystems.
      mask TypeOptions Port: Port
  Constant5 : Constant  Value=0  OutDataTypeStr=Inherit: Inherit via back propagation
  Logical Operator1 : Logic  Inputs=Inputs  AllPortsSameDT=off  OutDataTypeStr=boolean  mask(Logical Operator){Operator=AND, Inputs=2}
      mask prompts: Operator "Simulink:blkprm_prompts:LogicOperator"; Inputs "Simulink:blkprm_prompts:LogicNumInputPorts"
      mask help: Logical operators. For a single input, operators are applied across the input vector. For multiple inputs, operators are applied across the inputs.
      mask TypeOptions Operator: Operator
      mask TypeOptions Inputs: Inputs
  Relational Operator : RelationalOperator  Operator=<  OutDataTypeStr=boolean  RndMeth=Nearest  mask(Relational Operator){Operator=<}
      mask prompts: Operator "Simulink:blkprm_prompts:RelopOperator"
      mask help: Applies the selected relational operator to the inputs and outputs the result. The top (or left) input corresponds to the first operand.
      mask TypeOptions Operator: Operator
  Sum : Sum  InputSameDT=on  mask(Sum){Inputs=++}
      mask prompts: Inputs "Simulink:blkprm_prompts:SumListofSigns"
      mask help:
      | Add or subtract inputs.  Specify one of the following:
      | a) character vector containing + or - for each input port, | for spacer between ports (e.g. ++|-|++)
      | b) scalar, >= 1, specifies the number of input ports to be summed.
      | When there is only one input port, add or subtract elements over all dimensions or one specified dimension
      mask TypeOptions Inputs: Inputs
  Switch1 : Switch  Threshold=0.5  mask(Switch){}
      mask help: Pass through input 1 when input 2 satisfies the selected criterion; otherwise, pass through input 3. The inputs are numbered top to bottom (or left to right). The first and third input ports are data ports, and the second input port is the control port. The criteria for control port 2 are u2 >= Threshold (0.5).
  Unit Delay : UnitDelay  InitialCondition=InitialCondition  SampleTime=-1  mask(Unit Delay){InitialCondition=0}
      mask prompts: InitialCondition "Simulink:blkprm_prompts:DelayBlkInitCond"
      mask help: Sample and hold with one sample period delay.
      mask TypeOptions InitialCondition: InitialCondition
  hold_act : Outport  mask(Standard Outport){Port=1}
      mask prompts: Port "Simulink:blkprm_prompts:InOutportPortNum"
      mask help: Provide an output port for subsystems.
      mask TypeOptions Port: Port
  wires:
  Logical Operator1/1 -> hold_act/1
  Relational Operator/1 -> Logical Operator1/1
  Sum/1 -> Switch1/1
  Switch1/1 -> Unit Delay/1, Relational Operator/1
  condition/1 -> Switch1/2, Logical Operator1/2
  hold_t/1 -> Relational Operator/2
  Constant5/1 -> Switch1/3
  step_time/1 -> Sum/2
  Unit Delay/1 -> Sum/1
